simulink model "LIN_2DOF"  (R2019b)
settings: Solver=VariableStepAuto  StartTime=0.0  StopTime=10.0  RelTol=1e-3
InitFcn:
  | load("parameters.mat");
  | load("Coefficients.mat");
undefined symbols (not defined in the file): Dm, Dt, g, Jp, Jy, k_pitch, k_py, k_yaw, k_yp, Mb, w_neg_0, w_neg_1, w_pos_0, w_pos_1
libraries: cstblocks x3
settings Model: Creator=laptop  LastModifiedBy=lbend

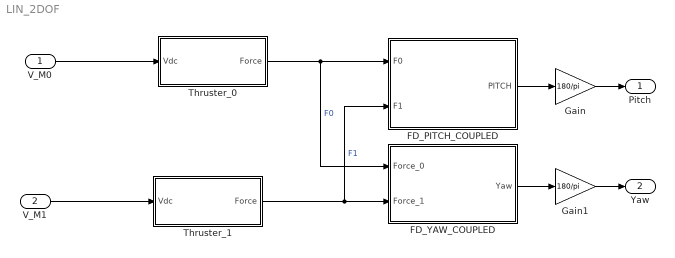
== system LIN_2DOF ==
  "V_M0 " : Inport
  "V_M1 " : Inport  Port=2
  FD_PITCH_COUPLED : Subsystem
  FD_YAW_COUPLED : Subsystem
  Gain : Gain  Gain=180/pi
  Gain1 : Gain  Gain=180/pi
  Thruster_0 : Subsystem
  "Thruster_1 " : Subsystem
  Pitch : Outport
  "Yaw " : Outport  Port=2
  wires:
  "V_M1 "/1 -> "Thruster_1 "/1(Vdc)
  Thruster_0/1(Force) -> FD_PITCH_COUPLED/1(F0), FD_YAW_COUPLED/1(Force_0)  "F0"
  "V_M0 "/1 -> Thruster_0/1(Vdc)
  "Thruster_1 "/1(Force) -> FD_PITCH_COUPLED/2(F1), FD_YAW_COUPLED/2(Force_1)  "F1"
  FD_PITCH_COUPLED/1(PITCH) -> Gain/1
  FD_YAW_COUPLED/1(Yaw) -> Gain1/1
  Gain/1 -> Pitch/1
  Gain1/1 -> "Yaw "/1

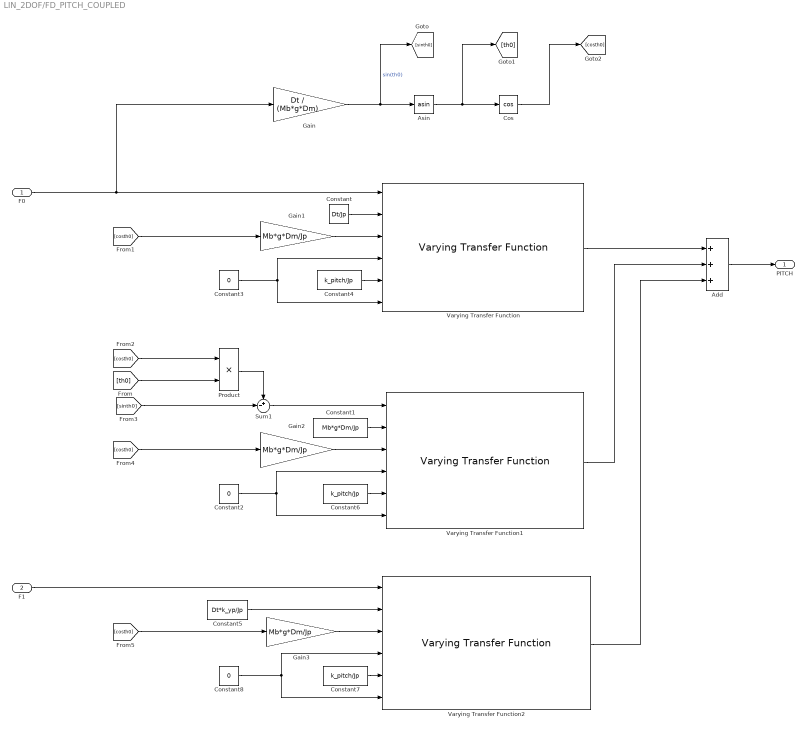
== system LIN_2DOF/FD_PITCH_COUPLED ==
  F0 : Inport
  F1 : Inport  Port=2
  Add : Sum  Inputs=+++
  Asin : Trigonometry  Operator=asin
  Constant : Constant  Value=Dt/Jp  SampleTime=0
  Constant1 : Constant  Value=Mb*g*Dm/Jp  SampleTime=0
  Constant2 : Constant  Value=0  SampleTime=0
  Constant3 : Constant  Value=0  SampleTime=0
  Constant4 : Constant  Value=k_pitch/Jp  SampleTime=0
  Constant5 : Constant  Value=Dt*k_yp/Jp  SampleTime=0
  Constant6 : Constant  Value=k_pitch/Jp  SampleTime=0
  Constant7 : Constant  Value=k_pitch/Jp  SampleTime=0
  Constant8 : Constant  Value=0  SampleTime=0
  Cos : Trigonometry  Operator=cos
  Gain : Gain  Gain=Dt / (Mb*g*Dm)
  Gain1 : Gain  Gain=Mb*g*Dm/Jp
  Gain2 : Gain  Gain=Mb*g*Dm/Jp
  Gain3 : Gain  Gain=Mb*g*Dm/Jp
  Product : Product
  Sum1 : Sum  Inputs=+-|
  Varying Transfer Function : cstblocks/Linear Parameter Varying/Varying Transfer Function  N=2
      settings: SourceProductName=Control System Toolbox
  Varying Transfer Function1 : cstblocks/Linear Parameter Varying/Varying Transfer Function  N=2
      settings: SourceProductName=Control System Toolbox
  Varying Transfer Function2 : cstblocks/Linear Parameter Varying/Varying Transfer Function  N=2
      settings: SourceProductName=Control System Toolbox
  PITCH : Outport
  wires:
  Constant8/1 -> Varying Transfer Function2/4, Varying Transfer Function2/6
  Cos/1 -> [costh0]
  Constant3/1 -> Varying Transfer Function/4, Varying Transfer Function/6
  Gain2/1 -> Varying Transfer Function1/3
  Varying Transfer Function2/1 -> Add/3
  Asin/1 -> Cos/1, [th0]
  Constant7/1 -> Varying Transfer Function2/5
  Constant1/1 -> Varying Transfer Function1/2
  Constant2/1 -> Varying Transfer Function1/4, Varying Transfer Function1/6
  Constant6/1 -> Varying Transfer Function1/5
  Gain/1 -> [sinth0], Asin/1  "sin(th0)"
  [costh0] -> Gain1/1
  [th0] -> Product/2
  [costh0] -> Product/1
  Constant4/1 -> Varying Transfer Function/5
  F0/1 -> Varying Transfer Function/1, Gain/1
  [sinth0] -> Sum1/2
  Product/1 -> Sum1/1
  [costh0] -> Gain2/1
  Varying Transfer Function/1 -> Add/1
  Varying Transfer Function1/1 -> Add/2
  Gain1/1 -> Varying Transfer Function/3
  Sum1/1 -> Varying Transfer Function1/1
  Constant5/1 -> Varying Transfer Function2/2
  Constant/1 -> Varying Transfer Function/2
  [costh0] -> Gain3/1
  Add/1 -> PITCH/1
  Gain3/1 -> Varying Transfer Function2/3
  F1/1 -> Varying Transfer Function2/1

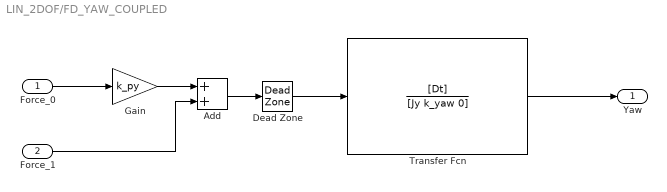
== system LIN_2DOF/FD_YAW_COUPLED ==
  Force_0 : Inport
  Force_1 : Inport  Port=2
  Add : Sum
  Dead Zone : DeadZone  LowerValue=F_limit_yaw  UpperValue=F_limit_yaw  SaturateOnIntegerOverflow=on
  Gain : Gain  Gain=k_py
  Transfer Fcn : TransferFcn  Numerator=[Dt]  Denominator=[Jy k_yaw 0]
  Yaw : Outport
  wires:
  Transfer Fcn/1 -> Yaw/1
  Dead Zone/1 -> Transfer Fcn/1
  Force_0/1 -> Gain/1
  Add/1 -> Dead Zone/1
  Gain/1 -> Add/1
  Force_1/1 -> Add/2

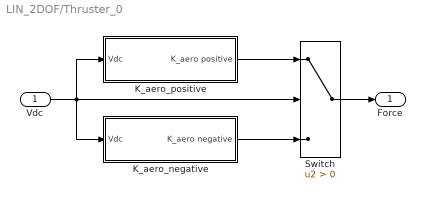
== system LIN_2DOF/Thruster_0 ==
  Vdc : Inport
  K_aero_negative : Subsystem
  K_aero_positive : Subsystem
  Switch : Switch  Criteria=u2 > Threshold
  Force : Outport
  wires:
  Switch/1 -> Force/1
  K_aero_positive/1(K_aero positive) -> Switch/1
  Vdc/1 -> K_aero_positive/1(Vdc), K_aero_negative/1(Vdc), Switch/2
  K_aero_negative/1(K_aero negative) -> Switch/3

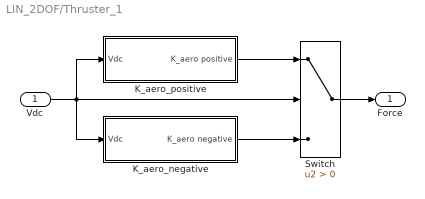
== system LIN_2DOF/Thruster_1  ==
  Vdc : Inport
  K_aero_negative : Subsystem
  K_aero_positive : Subsystem
  Switch : Switch  Criteria=u2 > Threshold
  Force : Outport
  wires:
  Switch/1 -> Force/1
  K_aero_positive/1(K_aero positive) -> Switch/1
  Vdc/1 -> K_aero_negative/1(Vdc), Switch/2, K_aero_positive/1(Vdc)
  K_aero_negative/1(K_aero negative) -> Switch/3

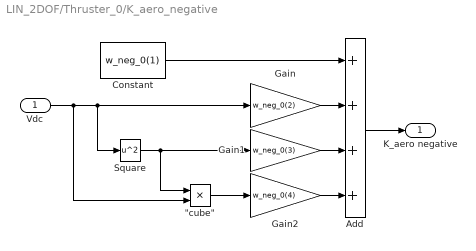
== system LIN_2DOF/Thruster_0/K_aero_negative ==
  Vdc : Inport
  "\"cube\"" : Product  Inputs=**
  Add : Sum  Inputs=++++
  Constant : Constant  Value=w_neg_0(1)  SampleTime=0
  Gain : Gain  Gain=w_neg_0(2)
  Gain1 : Gain  Gain=w_neg_0(3)
  Gain2 : Gain  Gain=w_neg_0(4)
  Square : Math  Operator=square  SignedPower=off  SaturateOnIntegerOverflow=on
  K_aero negative : Outport
  wires:
  Constant/1 -> Add/1
  Vdc/1 -> "\"cube\""/2, Square/1, Gain/1
  Add/1 -> K_aero negative/1
  Gain/1 -> Add/2
  Square/1 -> "\"cube\""/1, Gain1/1
  Gain1/1 -> Add/3
  Gain2/1 -> Add/4
  "\"cube\""/1 -> Gain2/1

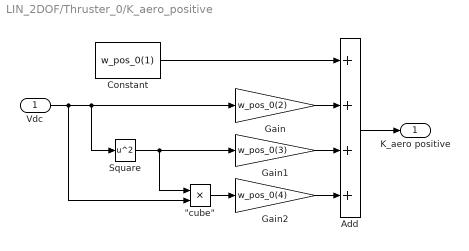
== system LIN_2DOF/Thruster_0/K_aero_positive ==
  Vdc : Inport
  "\"cube\"" : Product  Inputs=**
  Add : Sum  Inputs=++++
  Constant : Constant  Value=w_pos_0(1)  SampleTime=0
  Gain : Gain  Gain=w_pos_0(2)
  Gain1 : Gain  Gain=w_pos_0(3)
  Gain2 : Gain  Gain=w_pos_0(4)
  Square : Math  Operator=square  SignedPower=off  SaturateOnIntegerOverflow=on
  K_aero positive : Outport
  wires:
  Constant/1 -> Add/1
  Vdc/1 -> Gain/1, Square/1, "\"cube\""/2
  Add/1 -> K_aero positive/1
  Gain/1 -> Add/2
  Square/1 -> "\"cube\""/1, Gain1/1
  Gain1/1 -> Add/3
  "\"cube\""/1 -> Gain2/1
  Gain2/1 -> Add/4

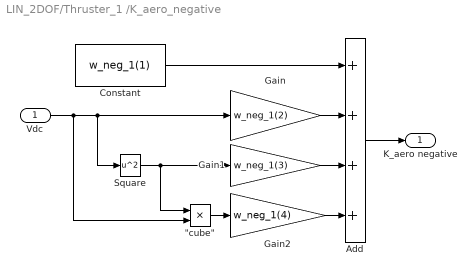
== system LIN_2DOF/Thruster_1 /K_aero_negative ==
  Vdc : Inport
  "\"cube\"" : Product  Inputs=**
  Add : Sum  Inputs=++++
  Constant : Constant  Value=w_neg_1(1)  SampleTime=0
  Gain : Gain  Gain=w_neg_1(2)
  Gain1 : Gain  Gain=w_neg_1(3)
  Gain2 : Gain  Gain=w_neg_1(4)
  Square : Math  Operator=square  SignedPower=off  SaturateOnIntegerOverflow=on
  K_aero negative : Outport
  wires:
  Constant/1 -> Add/1
  Vdc/1 -> "\"cube\""/2, Square/1, Gain/1
  Add/1 -> K_aero negative/1
  Gain/1 -> Add/2
  Square/1 -> "\"cube\""/1, Gain1/1
  Gain1/1 -> Add/3
  Gain2/1 -> Add/4
  "\"cube\""/1 -> Gain2/1

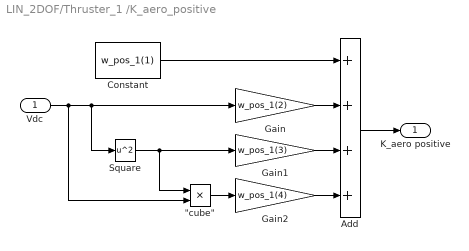
== system LIN_2DOF/Thruster_1 /K_aero_positive ==
  Vdc : Inport
  "\"cube\"" : Product  Inputs=**
  Add : Sum  Inputs=++++
  Constant : Constant  Value=w_pos_1(1)  SampleTime=0
  Gain : Gain  Gain=w_pos_1(2)
  Gain1 : Gain  Gain=w_pos_1(3)
  Gain2 : Gain  Gain=w_pos_1(4)
  Square : Math  Operator=square  SignedPower=off  SaturateOnIntegerOverflow=on
  K_aero positive : Outport
  wires:
  Constant/1 -> Add/1
  Vdc/1 -> Gain/1, Square/1, "\"cube\""/2
  Add/1 -> K_aero positive/1
  Gain/1 -> Add/2
  Square/1 -> "\"cube\""/1, Gain1/1
  Gain1/1 -> Add/3
  "\"cube\""/1 -> Gain2/1
  Gain2/1 -> Add/4
